simulink model "PassStBkReclnIsPosChk"  (R2018b)
settings: Solver=FixedStepDiscrete  StartTime=0.0  StopTime=10.0  RelTol=1e-3
undefined symbols (not defined in the file or in its folder): KeSMSuFirstRwStBackPosDelta_Val, KeSMSuFirstRwStBackPosTolr_Val
settings Model: Creator=sn2xws  LastModifiedBy=sn2xws
settings Model: ModifiedHistory=|
  | 2024.7.5 V3.0.0 557 模式流程V1.9
  | 2024.8.14 V3.0.1 NotMovFlg从库函数中移出
settings DataIOCC: SaveFormat=StructureWithTime
settings OptimizationCC: DefaultParameterBehavior=Inlined  EnhancedBackFolding=on  PassReuseOutputArgsAs=Individual arguments  ZeroExternalMemoryAtStartup=off  ZeroInternalMemoryAtStartup=off  OptimizeBlockOrder=speed  DifferentSizesBufferReuse=on  OptimizationCustomize=off
settings DebuggingCC: ParameterTunabilityLossMsg=error
settings SFSimCC: MATLABDynamicMemAlloc=off
settings RTWCC: SystemTargetFile=autosar.tlc  GenCodeOnly=on  TemplateMakefile=ert_default_tmf  Description=AUTOSAR  GenerateReport=on  IncludeHyperlinkInReport=on  LaunchReport=on  GenerateTraceInfo=on  GenerateTraceReport=on  GenerateTraceReportSl=on  GenerateTraceReportSf=on  GenerateTraceReportEml=on
settings CodeAppCC: ForceParamTrailComments=on  IgnoreCustomStorageClasses=off  OperatorAnnotations=on  SimulinkDataObjDesc=on  SFDataObjDesc=on  InsertBlockDesc=on
settings STFCustomTargetCC: TargetLangStandard=C99 (ISO)  MultiwordLength=256  ParMdlRefBuildCompliant=on  CompOptLevelCompliant=on  IncludeMdlTerminateFcn=off  CombineOutputUpdateFcns=on  SuppressErrorStatus=on  ERTCustomFileBanners=on  SupportNonFinite=off  SupportComplex=off  SupportContinuousTime=off  SupportNonInlinedSFcns=off  RemoveResetFunc=on  MATLABClassNameForMDSCustomization=Simulink.SoftwareTarget.ERTCustomization  AutosarCompliant=on  UseToolchainInfoCompliant=on  LookupTableObjectStructAxisOrder=2,1,3,4,...  LUTObjectStructOrderEvenSpacing=Size,Table,Breakpoints  SystemTargetFile=autosar.tlc
settings ERTTargetCC: TargetLangStandard=C99 (ISO)  ConcurrentExecutionCompliant=off  IncludeMdlTerminateFcn=off  SuppressErrorStatus=on  SupportNonFinite=off  SupportComplex=off  ModelStepFunctionPrototypeControlCompliant=off  CPPClassGenCompliant=off  AutosarCompliant=on  LookupTableObjectStructAxisOrder=2,1,3,4,...  LUTObjectStructOrderEvenSpacing=Size,Table,Breakpoints  InlinedParameterPlacement=NonHierarchical  ERTCustomFileTemplate=example_file_process.tlc  ERTFilePackagingFormat=Compact

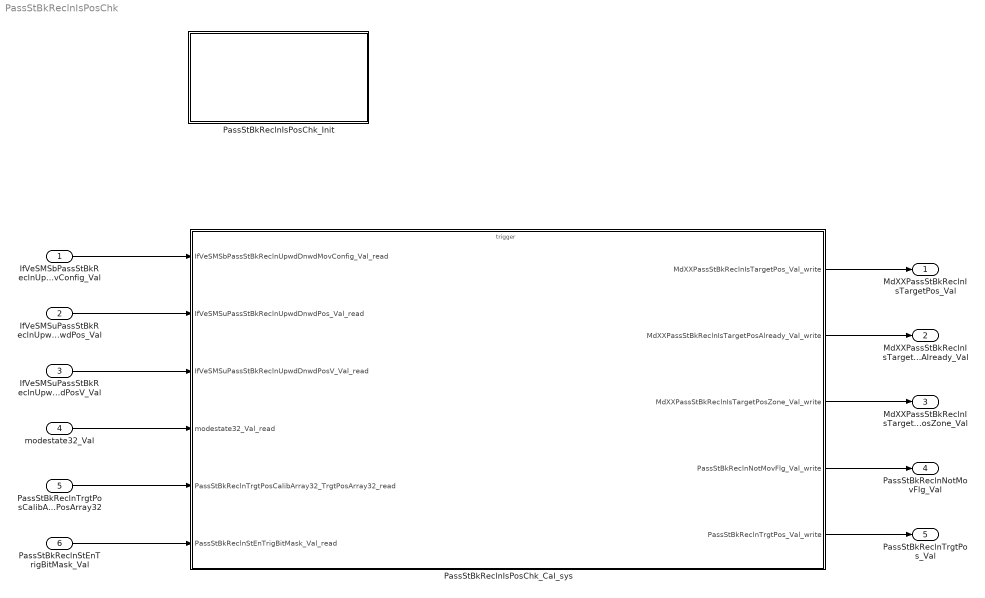
== system PassStBkReclnIsPosChk ==
  IfVeSMSbPassStBkReclnUpwdDnwdMovConfig_Val : Inport  OutDataTypeStr=boolean  PortDimensions=1
  IfVeSMSuPassStBkReclnUpwdDnwdPos_Val : Inport  Port=2  OutDataTypeStr=uint16  PortDimensions=1
  IfVeSMSuPassStBkReclnUpwdDnwdPosV_Val : Inport  Port=3  OutDataTypeStr=boolean  PortDimensions=1
  modestate32_Val : Inport  Port=4  OutDataTypeStr=uint32  PortDimensions=1
  PassStBkReclnTrgtPosCalibArray32_TrgtPosArray32 : Inport  Description=|  Port=5  OutDataTypeStr=uint16  PortDimensions=96
      | 0:Pos
      | 1:Max
      | 2:Min
  PassStBkReclnStEnTrigBitMask_Val : Inport  Port=6  OutDataTypeStr=uint32  PortDimensions=1
  PassStBkReclnIsPosChk_Cal_sys : Subsystem
  PassStBkReclnIsPosChk_Init : Subsystem
  MdXXPassStBkReclnIsTargetPos_Val : Outport  OutDataTypeStr=uint32  PortDimensions=1
  MdXXPassStBkReclnIsTargetPosAlready_Val : Outport  Port=2  OutDataTypeStr=uint32  PortDimensions=1
  MdXXPassStBkReclnIsTargetPosZone_Val : Outport  Port=3  OutDataTypeStr=uint32  PortDimensions=1
  PassStBkReclnNotMovFlg_Val : Outport  Port=4  OutDataTypeStr=boolean  PortDimensions=1
  PassStBkReclnTrgtPos_Val : Outport  Port=5  OutDataTypeStr=uint16  PortDimensions=1
  wires:
  IfVeSMSbPassStBkReclnUpwdDnwdMovConfig_Val/1 -> PassStBkReclnIsPosChk_Cal_sys/1(IfVeSMSbPassStBkReclnUpwdDnwdMovConfig_Val_read)
  IfVeSMSuPassStBkReclnUpwdDnwdPos_Val/1 -> PassStBkReclnIsPosChk_Cal_sys/2(IfVeSMSuPassStBkReclnUpwdDnwdPos_Val_read)
  IfVeSMSuPassStBkReclnUpwdDnwdPosV_Val/1 -> PassStBkReclnIsPosChk_Cal_sys/3(IfVeSMSuPassStBkReclnUpwdDnwdPosV_Val_read)
  modestate32_Val/1 -> PassStBkReclnIsPosChk_Cal_sys/4(modestate32_Val_read)
  PassStBkReclnTrgtPosCalibArray32_TrgtPosArray32/1 -> PassStBkReclnIsPosChk_Cal_sys/5(PassStBkReclnTrgtPosCalibArray32_TrgtPosArray32_read)
  PassStBkReclnIsPosChk_Cal_sys/1(MdXXPassStBkReclnIsTargetPos_Val_write) -> MdXXPassStBkReclnIsTargetPos_Val/1
  PassStBkReclnIsPosChk_Cal_sys/2(MdXXPassStBkReclnIsTargetPosAlready_Val_write) -> MdXXPassStBkReclnIsTargetPosAlready_Val/1
  PassStBkReclnIsPosChk_Cal_sys/3(MdXXPassStBkReclnIsTargetPosZone_Val_write) -> MdXXPassStBkReclnIsTargetPosZone_Val/1
  PassStBkReclnIsPosChk_Cal_sys/4(PassStBkReclnNotMovFlg_Val_write) -> PassStBkReclnNotMovFlg_Val/1
  PassStBkReclnIsPosChk_Cal_sys/5(PassStBkReclnTrgtPos_Val_write) -> PassStBkReclnTrgtPos_Val/1
  PassStBkReclnStEnTrigBitMask_Val/1 -> PassStBkReclnIsPosChk_Cal_sys/6(PassStBkReclnStEnTrigBitMask_Val_read)

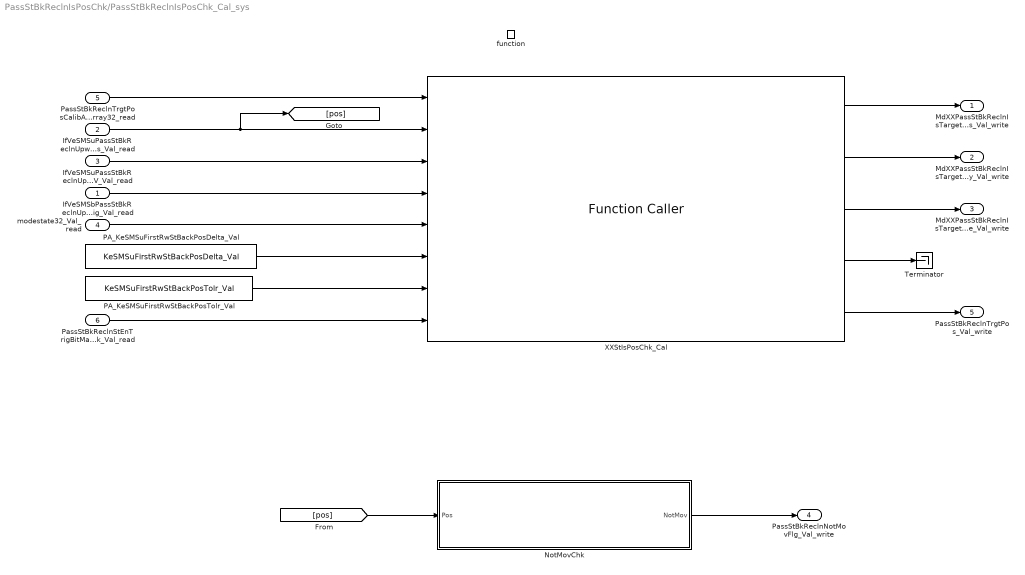
== system PassStBkReclnIsPosChk/PassStBkReclnIsPosChk_Cal_sys ==
  IfVeSMSbPassStBkReclnUpwdDnwdMovConfig_Val_read : Inport
  IfVeSMSuPassStBkReclnUpwdDnwdPos_Val_read : Inport  Port=2
  IfVeSMSuPassStBkReclnUpwdDnwdPosV_Val_read : Inport  Port=3
  modestate32_Val_read : Inport  Port=4
  PassStBkReclnTrgtPosCalibArray32_TrgtPosArray32_read : Inport  Port=5
  PassStBkReclnStEnTrigBitMask_Val_read : Inport  Port=6
  function : TriggerPort  TriggerType=function-call  IsSimulinkFunction=on  FunctionName=PassStBkReclnIsPosChk_Cal  VariantControl=(inherit)
  NotMovChk : Subsystem
  PA_KeSMSuFirstRwStBackPosDelta_Val : Constant  Value=KeSMSuFirstRwStBackPosDelta_Val
  PA_KeSMSuFirstRwStBackPosTolr_Val : Constant  Value=KeSMSuFirstRwStBackPosTolr_Val
  Terminator : Terminator
  XXStIsPosChk_Cal : FunctionCaller  FunctionPrototype=[IsPos,IsPosAlready,IsPosZone,NotMovFlg,StTrgtPos] = XXStIsPosChk_Cal(MdCalibArray32,Pos,PosV,MovConfig,modestate32,PosDelta,PosTolr,StBitMask)  InputArgumentSpecifications=uint16([1;1;1;1;1;1;1;1;1;1;1;1;1;1;1;1;1;1;1;1;1;1;1;1;1;1;1;1;1;1;1;1;1;1;1;1;1;1;1;1;1;1;1;1;1;1;1;1;1;1;1;1;1;1;1;1;1;1;1;1;1;1;1;1;1;1;1;1;1;1;1;1;1;1;1;1;1;1;1;1;1;1;1;1;1;1;1;1;1;1;1;1;1;1;1;1]), uint16(1), boolean(true), boolean(true), uint32(1), uint16(1), uint16(1), uint32(1)  OutputArgumentSpecifications=uint32(1), uint32(1), uint32(1), boolean(true), uint16(1)
  MdXXPassStBkReclnIsTargetPos_Val_write : Outport
      settings: EnsureOutportIsVirtual=on
  MdXXPassStBkReclnIsTargetPosAlready_Val_write : Outport  Port=2
      settings: EnsureOutportIsVirtual=on
  MdXXPassStBkReclnIsTargetPosZone_Val_write : Outport  Port=3
      settings: EnsureOutportIsVirtual=on
  PassStBkReclnNotMovFlg_Val_write : Outport  Port=4
      settings: EnsureOutportIsVirtual=on
  PassStBkReclnTrgtPos_Val_write : Outport  Port=5
      settings: EnsureOutportIsVirtual=on
  wires:
  XXStIsPosChk_Cal/2 -> MdXXPassStBkReclnIsTargetPosAlready_Val_write/1
  XXStIsPosChk_Cal/1 -> MdXXPassStBkReclnIsTargetPos_Val_write/1
  XXStIsPosChk_Cal/3 -> MdXXPassStBkReclnIsTargetPosZone_Val_write/1
  XXStIsPosChk_Cal/5 -> PassStBkReclnTrgtPos_Val_write/1
  IfVeSMSuPassStBkReclnUpwdDnwdPos_Val_read/1 -> [pos], XXStIsPosChk_Cal/2
  IfVeSMSuPassStBkReclnUpwdDnwdPosV_Val_read/1 -> XXStIsPosChk_Cal/3
  IfVeSMSbPassStBkReclnUpwdDnwdMovConfig_Val_read/1 -> XXStIsPosChk_Cal/4
  modestate32_Val_read/1 -> XXStIsPosChk_Cal/5
  PA_KeSMSuFirstRwStBackPosDelta_Val/1 -> XXStIsPosChk_Cal/6
  PA_KeSMSuFirstRwStBackPosTolr_Val/1 -> XXStIsPosChk_Cal/7
  PassStBkReclnTrgtPosCalibArray32_TrgtPosArray32_read/1 -> XXStIsPosChk_Cal/1
  PassStBkReclnStEnTrigBitMask_Val_read/1 -> XXStIsPosChk_Cal/8
  [pos] -> NotMovChk/1(Pos)
  NotMovChk/1(NotMov) -> PassStBkReclnNotMovFlg_Val_write/1
  XXStIsPosChk_Cal/4 -> Terminator/1

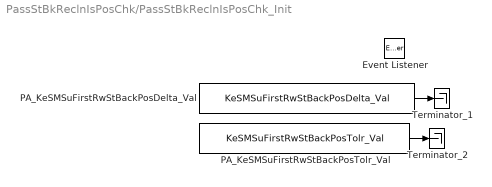
== system PassStBkReclnIsPosChk/PassStBkReclnIsPosChk_Init ==
  Event Listener : EventListener  EventName=reset
  PA_KeSMSuFirstRwStBackPosDelta_Val : Constant  Value=KeSMSuFirstRwStBackPosDelta_Val
  PA_KeSMSuFirstRwStBackPosTolr_Val : Constant  Value=KeSMSuFirstRwStBackPosTolr_Val
  Terminator_1 : Terminator
  Terminator_2 : Terminator
  wires:
  PA_KeSMSuFirstRwStBackPosDelta_Val/1 -> Terminator_1/1
  PA_KeSMSuFirstRwStBackPosTolr_Val/1 -> Terminator_2/1

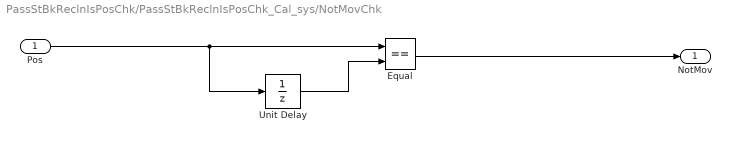
== system PassStBkReclnIsPosChk/PassStBkReclnIsPosChk_Cal_sys/NotMovChk ==
  Pos : Inport
  Equal : RelationalOperator  Operator===  OutDataTypeStr=boolean  RndMeth=Simplest
  Unit Delay : UnitDelay  SampleTime=-1
  NotMov : Outport
  wires:
  Unit Delay/1 -> Equal/2
  Pos/1 -> Unit Delay/1, Equal/1
  Equal/1 -> NotMov/1
